simulink model "w1p9"  (R2020b)
settings: Solver=VariableStepAuto  StartTime=0.0  StopTime=10.0  RelTol=1e-3
model workspace (MAT data in the model file):
  B = 1e-06
  J = 1.517e-05
  Ke = 5.623e-05
  L = 0.00505
  P = 4
  R = 4.98
  Sig = Simulink.Signal
  Sig.DataType = 'auto'
  Sig.Dimensions = -1
  Sig.DimensionsMode = 'auto'
  Sig.Complexity = 'auto'
  Sig.SampleTime = -1
  Sig.SamplingMode = 'auto'
  Tm = 0.1
settings Model: Creator=family  LastModifiedBy=family

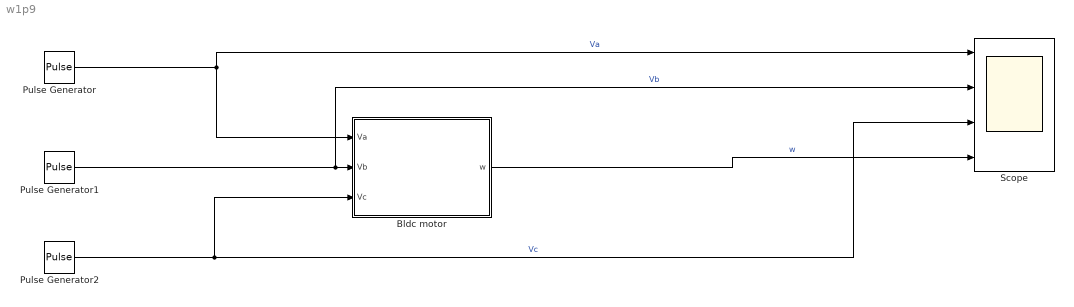
== system w1p9 ==
  Bldc motor : Subsystem
  Pulse Generator : DiscretePulseGenerator  PulseType=Time based  Amplitude=30  Period=10  PulseWidth=30
  Pulse Generator1 : DiscretePulseGenerator  PulseType=Time based  Amplitude=30  Period=10  PulseWidth=30  PhaseDelay=2.8
  Pulse Generator2 : DiscretePulseGenerator  PulseType=Time based  Amplitude=30  Period=10  PulseWidth=30  PhaseDelay=5.8
  Scope : Scope  NumInputPorts=4
  wires:
  Pulse Generator1/1 -> Scope/2, Bldc motor/2(Vb)  "Vb"
  Pulse Generator2/1 -> Scope/3, Bldc motor/3(Vc)  "Vc"
  Bldc motor/1(w) -> Scope/4  "w"
  Pulse Generator/1 -> Bldc motor/1(Va), Scope/1  "Va"

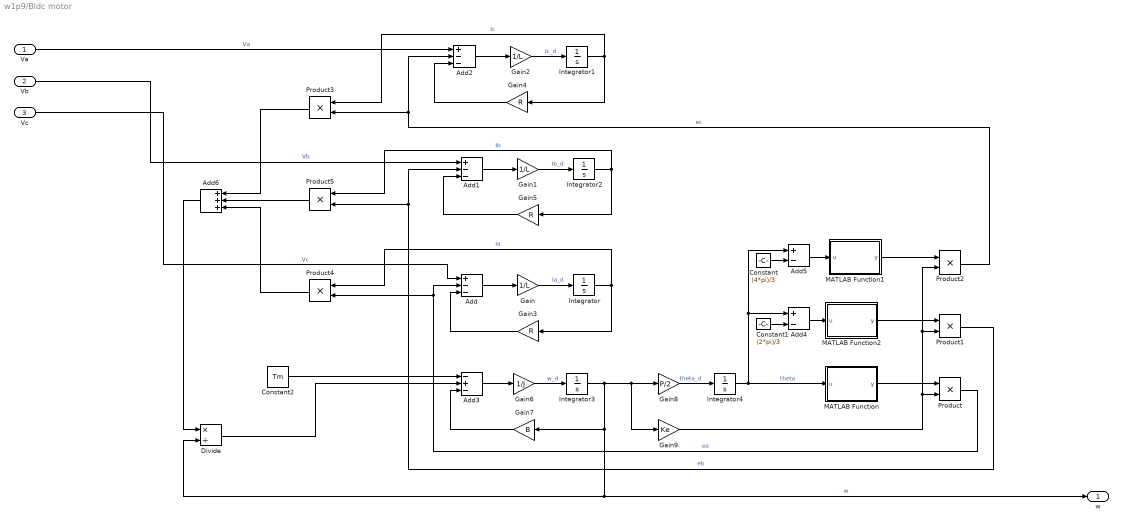
== system w1p9/Bldc motor ==
  Va : Inport
  Vb : Inport  Port=2
  Vc : Inport  Port=3
  Add : Sum  Inputs=+--
  Add1 : Sum  Inputs=+--
  Add2 : Sum  Inputs=+--
  Add3 : Sum  Inputs=-+-
  Add4 : Sum  Inputs=+-
  Add5 : Sum  Inputs=+-
  Add6 : Sum  Inputs=+++
  Constant : Constant  Value=(4*pi)/3
  Constant1 : Constant  Value=(2*pi)/3
  Constant2 : Constant  Value=Tm
  Divide : Product  Inputs=*/
  Gain : Gain  Gain=1/L
  Gain1 : Gain  Gain=1/L
  Gain2 : Gain  Gain=1/L
  Gain3 : Gain  Gain=R
  Gain4 : Gain  Gain=R
  Gain5 : Gain  Gain=R
  Gain6 : Gain  Gain=1/J
  Gain7 : Gain  Gain=B
  Gain8 : Gain  Gain=P/2
  Gain9 : Gain  Gain=Ke
  Integrator{,1..2,4} (4 alike) : Integrator
  Integrator3 : Integrator  InitialCondition=1
  MATLAB Function : MATLAB Function  TreatAsAtomicUnit=on
  MATLAB Function1 : MATLAB Function  TreatAsAtomicUnit=on
  MATLAB Function2 : MATLAB Function  TreatAsAtomicUnit=on
  Product{,1..5} (6 alike) : Product
  w : Outport
  wires:
  Gain9/1 -> Product2/2, Product1/2, Product/2
  Gain1/1 -> Integrator2/1  "Ib_d"
  Integrator/1 -> Gain3/1, Product4/1  "Ia"
  Integrator2/1 -> Gain5/1, Product5/1  "Ib"
  Integrator3/1 -> Gain8/1, Gain9/1, Gain7/1, w/1, Divide/2  "w"
  Add5/1 -> MATLAB Function1/1(u)
  Gain/1 -> Integrator/1  "Ia_d"
  MATLAB Function1/1(y) -> Product2/1
  Add2/1 -> Gain2/1
  Product2/1 -> Add2/2, Product3/2  "ec"
  Vc/1 -> Add/1  "Vc"
  Gain3/1 -> Add/3
  Product5/1 -> Add6/2
  Integrator1/1 -> Gain4/1, Product3/1  "Ic"
  Gain5/1 -> Add1/3
  Integrator4/1 -> MATLAB Function/1(u), Add5/1, Add4/1  "theta"
  Add/1 -> Gain/1
  Add3/1 -> Gain6/1
  Gain2/1 -> Integrator1/1  "Ic_d"
  Add6/1 -> Divide/1
  Constant1/1 -> Add4/2
  Constant/1 -> Add5/2
  MATLAB Function2/1(y) -> Product1/1
  Gain7/1 -> Add3/3
  Product4/1 -> Add6/3
  Gain6/1 -> Integrator3/1  "w_d"
  Va/1 -> Add2/1  "Va"
  Gain8/1 -> Integrator4/1  "theta_d"
  MATLAB Function/1(y) -> Product/1
  Product/1 -> Product4/2, Add/2  "ea"
  Product1/1 -> Product5/2, Add1/2  "eb"
  Divide/1 -> Add3/2
  Gain4/1 -> Add2/3
  Add1/1 -> Gain1/1
  Product3/1 -> Add6/1
  Constant2/1 -> Add3/1
  Add4/1 -> MATLAB Function2/1(u)
  Vb/1 -> Add1/1  "Vb"

== matlab function w1p9/Bldc motor/MATLAB Function ==
  data: u input; y output
function y = fcn(u)

if (u>=0 && u<((2*pi)/3))
    y = 1;
elseif(u>=((2*pi)/3) && u<pi)
    y = 1-(6/pi*(u-((2*pi)/3)));
elseif(u>=pi && u<((5*pi)/3))
    y = -1;
else
    y = -1+(6/pi*(u-((5*pi)/3)));
end
end

== matlab function w1p9/Bldc motor/MATLAB Function2 ==
  data: u input; y output
function y = fcn(u)

if (u>=0 && u<((2*pi)/3))
    y = 1;
elseif(u>=((2*pi)/3) && u<pi)
    y = 1-(6/pi*(u-((2*pi)/3)));
elseif(u>=pi && u<((5*pi)/3))
    y = -1;
else
    y = -1+(6/pi*(u-((5*pi)/3)));
end
end

== matlab function w1p9/Bldc motor/MATLAB Function1 ==
  data: u input; y output
function y = fcn(u)

if (u>=0 && u<((2*pi)/3))
    y = 1;
elseif(u>=((2*pi)/3) && u<pi)
    y = 1-(6/pi*(u-((2*pi)/3)));
elseif(u>=pi && u<((5*pi)/3))
    y = -1;
else
    y = -1+(6/pi*(u-((5*pi)/3)));
end
end
